simulink model "Fly_By_Wire_Functional_Architecture"  (R2024b)
settings: Solver=VariableStepAuto  StartTime=0.0  StopTime=10.0  RelTol=1e-3
settings Model: Creator=kmara  LastModifiedBy=annicenajafi

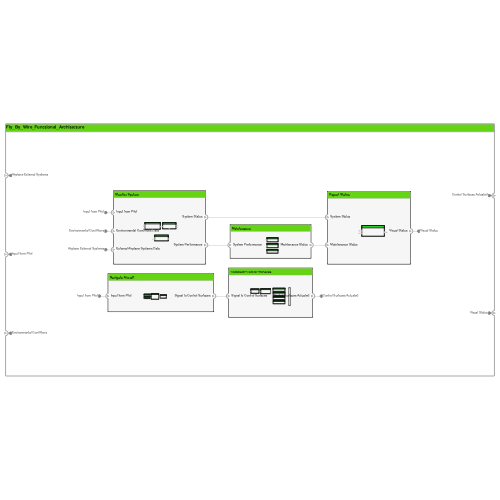
[thumbnail: Simulink's stored preview of the top-level diagram]
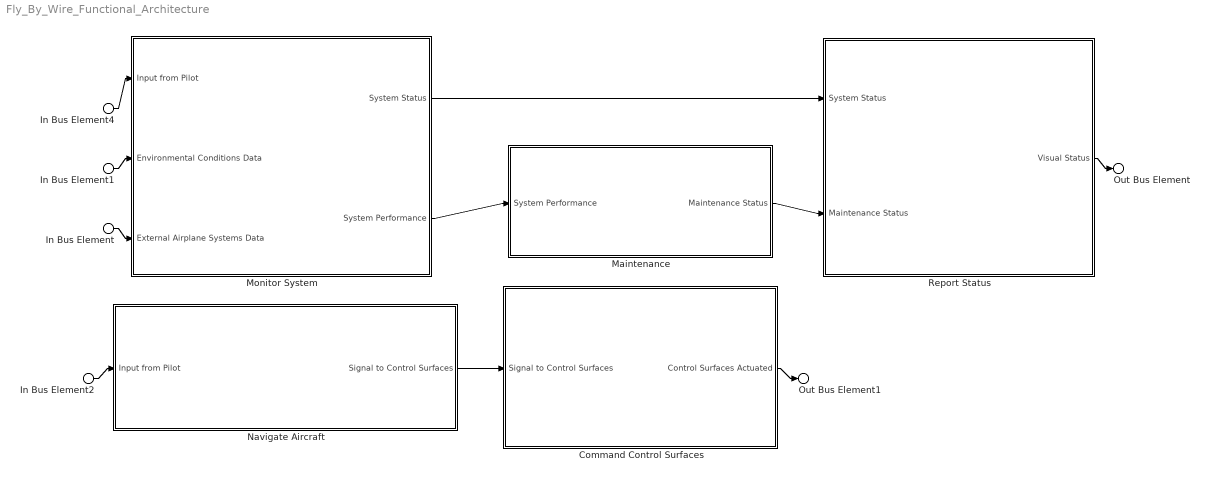
== system Fly_By_Wire_Functional_Architecture ==
  In Bus Element : Inport  PortName=Airplane External Systems
  In Bus Element2 : Inport  Port=2  PortName=Input from Pilot
  In Bus Element4 : Inport  Port=2  PortName=Input from Pilot
  In Bus Element1 : Inport  Port=3  PortName=Environmental Conditions
  Command Control Surfaces : Subsystem
      settings: PortSchema="{\"entries\":[{\"content\":{\"headerSize\":26,\"margin\":15,\"minimumSpacing\":25,\"sides\":[{\"content\":{\"connectorIds\":[\"In1\"]},\"type\":\"ConnectorPlacement.EquallySpacedRectSide\",\"uuid\":\"b623a921-0a01-4933-aa95-d281e4fd472d\"},{\"content\":{\"connectorIds\":[\"Out1\"],\"side\":\"RIGHT\"},\"type\":\"ConnectorPlacement.EquallySpacedRectSide\",\"uuid\":\"7949cc00-59a5-498d-8900-6268840cf223\"},{\"content\":{\"side\":\"TOP\"},\"type\":\"ConnectorPlacement.EquallySpacedRectSide\",\"uuid\":\"61a6df68-b8b8-47cf-a694-eae6da7c16c5\"}]},\"type\":\"ConnectorPlacement.EquallySpacedConnector\",\"uuid\":\"95d0e082-c8fd-4f2c-a7f4-dd74223482be\"}],\"packageUris\":[\"http://schema.mathworks.com/mf0/Connector/R2020b\"],\"version\":\"1.0\"}"
  Maintenance : Subsystem
      settings: PortSchema="{\"entries\":[{\"content\":{\"headerSize\":26,\"margin\":15,\"minimumSpacing\":25,\"sides\":[{\"content\":{\"connectorIds\":[\"In1\"]},\"type\":\"ConnectorPlacement.EquallySpacedRectSide\",\"uuid\":\"b623a921-0a01-4933-aa95-d281e4fd472d\"},{\"content\":{\"connectorIds\":[\"Out1\"],\"side\":\"RIGHT\"},\"type\":\"ConnectorPlacement.EquallySpacedRectSide\",\"uuid\":\"7949cc00-59a5-498d-8900-6268840cf223\"},{\"content\":{\"side\":\"TOP\"},\"type\":\"ConnectorPlacement.EquallySpacedRectSide\",\"uuid\":\"61a6df68-b8b8-47cf-a694-eae6da7c16c5\"},{\"content\":{\"side\":\"BOTTOM\"},\"type\":\"ConnectorPlacement.EquallySpacedRectSide\",\"uuid\":\"116ec3ef-5420-49c5-b776-94fc19793a99\"}]},\"type\":\"ConnectorPlacement.EquallySpacedConnector\",\"uuid\":\"95d0e082-c8fd-4f2c-a7f4-dd74223482be\"}],\"packageUris\":[\"http://schema.mathworks.com/mf0/Connector/R2020b\"],\"version\":\"1.0\"}"
  Monitor System : Subsystem
      settings: PortSchema="{\"entries\":[{\"content\":{\"headerSize\":26,\"margin\":15,\"minimumSpacing\":25,\"sides\":[{\"content\":{\"connectorIds\":[\"In1\",\"In2\",\"In3\"]},\"type\":\"ConnectorPlacement.EquallySpacedRectSide\",\"uuid\":\"ca232a45-352c-4197-a2f1-cf960b1c61e1\"},{\"content\":{\"connectorIds\":[\"Out2\",\"Out1\"],\"side\":\"RIGHT\"},\"type\":\"ConnectorPlacement.EquallySpacedRectSide\",\"uuid\":\"283c5dac-edd1-4fd8-b197-00019376217d\"},{\"content\":{\"side\":\"TOP\"},\"type\":\"ConnectorPlacement.EquallySpacedRectSide\",\"uuid\":\"42446a2b-1c27-4301-a80a-90130219a089\"},{\"content\":{\"side\":\"BOTTOM\"},\"type\":\"ConnectorPlacement.EquallySpacedRectSide\",\"uuid\":\"c57680a4-00c2-4754-bdc7-f63d5f759134\"}]},\"type\":\"ConnectorPlacement.EquallySpacedConnector\",\"uuid\":\"458bc52f-ed05-4f31-b732-8171eb2e03be\"}],\"packageUris\":[\"http://schema.mathworks.com/mf0/Connector/R2020b\"],\"version\":\"1.0\"}"
  Navigate Aircraft : Subsystem
      settings: PortSchema="{\"entries\":[{\"content\":{\"headerSize\":26,\"margin\":15,\"minimumSpacing\":25,\"sides\":[{\"content\":{\"connectorIds\":[\"In1\"]},\"type\":\"ConnectorPlacement.EquallySpacedRectSide\",\"uuid\":\"b623a921-0a01-4933-aa95-d281e4fd472d\"},{\"content\":{\"connectorIds\":[\"Out1\"],\"side\":\"RIGHT\"},\"type\":\"ConnectorPlacement.EquallySpacedRectSide\",\"uuid\":\"7949cc00-59a5-498d-8900-6268840cf223\"},{\"content\":{\"side\":\"TOP\"},\"type\":\"ConnectorPlacement.EquallySpacedRectSide\",\"uuid\":\"61a6df68-b8b8-47cf-a694-eae6da7c16c5\"}]},\"type\":\"ConnectorPlacement.EquallySpacedConnector\",\"uuid\":\"95d0e082-c8fd-4f2c-a7f4-dd74223482be\"}],\"packageUris\":[\"http://schema.mathworks.com/mf0/Connector/R2020b\"],\"version\":\"1.0\"}"
  Report Status : Subsystem
      settings: PortSchema="{\"entries\":[{\"content\":{\"headerSize\":26,\"margin\":15,\"minimumSpacing\":25,\"sides\":[{\"content\":{\"connectorIds\":[\"In2\",\"In1\"]},\"type\":\"ConnectorPlacement.EquallySpacedRectSide\",\"uuid\":\"ca232a45-352c-4197-a2f1-cf960b1c61e1\"},{\"content\":{\"connectorIds\":[\"Out1\"],\"side\":\"RIGHT\"},\"type\":\"ConnectorPlacement.EquallySpacedRectSide\",\"uuid\":\"283c5dac-edd1-4fd8-b197-00019376217d\"},{\"content\":{\"side\":\"TOP\"},\"type\":\"ConnectorPlacement.EquallySpacedRectSide\",\"uuid\":\"42446a2b-1c27-4301-a80a-90130219a089\"}]},\"type\":\"ConnectorPlacement.EquallySpacedConnector\",\"uuid\":\"458bc52f-ed05-4f31-b732-8171eb2e03be\"}],\"packageUris\":[\"http://schema.mathworks.com/mf0/Connector/R2020b\"],\"version\":\"1.0\"}"
  Out Bus Element1 : Outport  PortName=Control Surfaces Actuated
  Out Bus Element : Outport  Port=2  PortName=Visual Status
  wires:
  In Bus Element4/1 -> Monitor System/1(Input from Pilot)
  In Bus Element/1 -> Monitor System/3(External Airplane Systems Data)
  In Bus Element2/1 -> Navigate Aircraft/1(Input from Pilot)
  Navigate Aircraft/1(Signal to Control Surfaces) -> Command Control Surfaces/1(Signal to Control Surfaces)
  In Bus Element1/1 -> Monitor System/2(Environmental Conditions Data)
  Monitor System/1(System Performance) -> Maintenance/1(System Performance)
  Monitor System/2(System Status) -> Report Status/2(System Status)
  Maintenance/1(Maintenance Status) -> Report Status/1(Maintenance Status)
  Command Control Surfaces/1(Control Surfaces Actuated) -> Out Bus Element1/1
  Report Status/1(Visual Status) -> Out Bus Element/1

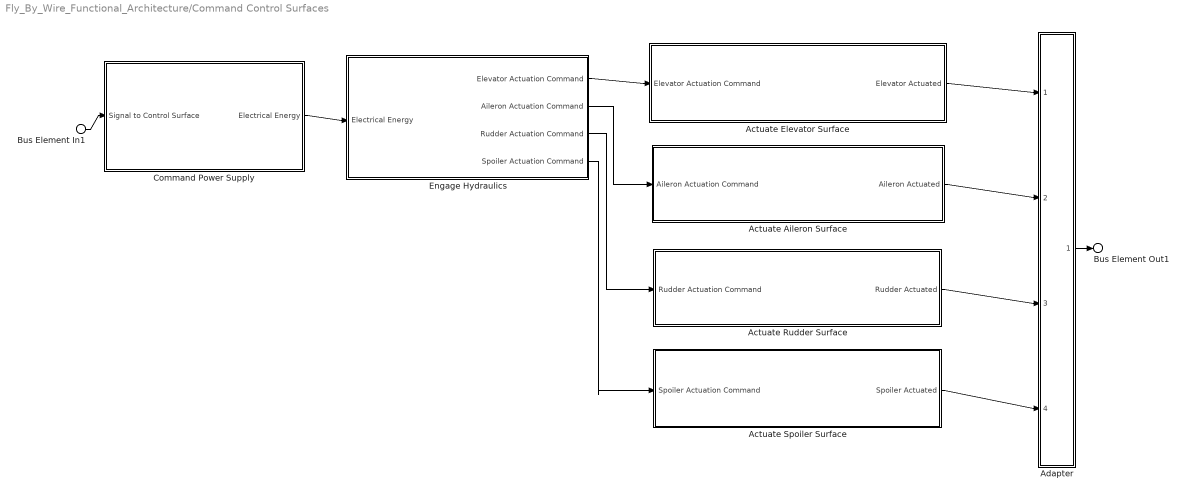
== system Fly_By_Wire_Functional_Architecture/Command Control Surfaces ==
  Bus Element In1 : Inport  PortName=Signal to Control Surfaces
  Actuate Aileron Surface : Subsystem
      settings: PortSchema="{\"entries\":[{\"content\":{\"headerSize\":26,\"margin\":15,\"minimumSpacing\":25,\"sides\":[{\"content\":{\"connectorIds\":[\"In1\"]},\"type\":\"ConnectorPlacement.EquallySpacedRectSide\",\"uuid\":\"b623a921-0a01-4933-aa95-d281e4fd472d\"},{\"content\":{\"connectorIds\":[\"Out1\"],\"side\":\"RIGHT\"},\"type\":\"ConnectorPlacement.EquallySpacedRectSide\",\"uuid\":\"7949cc00-59a5-498d-8900-6268840cf223\"},{\"content\":{\"side\":\"TOP\"},\"type\":\"ConnectorPlacement.EquallySpacedRectSide\",\"uuid\":\"61a6df68-b8b8-47cf-a694-eae6da7c16c5\"}]},\"type\":\"ConnectorPlacement.EquallySpacedConnector\",\"uuid\":\"95d0e082-c8fd-4f2c-a7f4-dd74223482be\"}],\"packageUris\":[\"http://schema.mathworks.com/mf0/Connector/R2020b\"],\"version\":\"1.0\"}"
  Actuate Elevator Surface : Subsystem
      settings: PortSchema="{\"entries\":[{\"content\":{\"headerSize\":26,\"margin\":15,\"minimumSpacing\":25,\"sides\":[{\"content\":{\"connectorIds\":[\"In1\"]},\"type\":\"ConnectorPlacement.EquallySpacedRectSide\",\"uuid\":\"b623a921-0a01-4933-aa95-d281e4fd472d\"},{\"content\":{\"connectorIds\":[\"Out1\"],\"side\":\"RIGHT\"},\"type\":\"ConnectorPlacement.EquallySpacedRectSide\",\"uuid\":\"7949cc00-59a5-498d-8900-6268840cf223\"},{\"content\":{\"side\":\"TOP\"},\"type\":\"ConnectorPlacement.EquallySpacedRectSide\",\"uuid\":\"61a6df68-b8b8-47cf-a694-eae6da7c16c5\"}]},\"type\":\"ConnectorPlacement.EquallySpacedConnector\",\"uuid\":\"95d0e082-c8fd-4f2c-a7f4-dd74223482be\"}],\"packageUris\":[\"http://schema.mathworks.com/mf0/Connector/R2020b\"],\"version\":\"1.0\"}"
  Actuate Rudder Surface : Subsystem
      settings: PortSchema="{\"entries\":[{\"content\":{\"headerSize\":26,\"margin\":15,\"minimumSpacing\":25,\"sides\":[{\"content\":{\"connectorIds\":[\"In1\"]},\"type\":\"ConnectorPlacement.EquallySpacedRectSide\",\"uuid\":\"b623a921-0a01-4933-aa95-d281e4fd472d\"},{\"content\":{\"connectorIds\":[\"Out1\"],\"side\":\"RIGHT\"},\"type\":\"ConnectorPlacement.EquallySpacedRectSide\",\"uuid\":\"7949cc00-59a5-498d-8900-6268840cf223\"},{\"content\":{\"side\":\"TOP\"},\"type\":\"ConnectorPlacement.EquallySpacedRectSide\",\"uuid\":\"61a6df68-b8b8-47cf-a694-eae6da7c16c5\"}]},\"type\":\"ConnectorPlacement.EquallySpacedConnector\",\"uuid\":\"95d0e082-c8fd-4f2c-a7f4-dd74223482be\"}],\"packageUris\":[\"http://schema.mathworks.com/mf0/Connector/R2020b\"],\"version\":\"1.0\"}"
  Actuate Spoiler Surface : Subsystem
      settings: PortSchema="{\"entries\":[{\"content\":{\"headerSize\":26,\"margin\":15,\"minimumSpacing\":25,\"sides\":[{\"content\":{\"connectorIds\":[\"In1\"]},\"type\":\"ConnectorPlacement.EquallySpacedRectSide\",\"uuid\":\"b623a921-0a01-4933-aa95-d281e4fd472d\"},{\"content\":{\"connectorIds\":[\"Out1\"],\"side\":\"RIGHT\"},\"type\":\"ConnectorPlacement.EquallySpacedRectSide\",\"uuid\":\"7949cc00-59a5-498d-8900-6268840cf223\"},{\"content\":{\"side\":\"TOP\"},\"type\":\"ConnectorPlacement.EquallySpacedRectSide\",\"uuid\":\"61a6df68-b8b8-47cf-a694-eae6da7c16c5\"}]},\"type\":\"ConnectorPlacement.EquallySpacedConnector\",\"uuid\":\"95d0e082-c8fd-4f2c-a7f4-dd74223482be\"}],\"packageUris\":[\"http://schema.mathworks.com/mf0/Connector/R2020b\"],\"version\":\"1.0\"}"
  Adapter : Subsystem
      settings: PortSchema="{\"entries\":[{\"content\":{\"margin\":10,\"minimumSpacing\":15,\"sides\":[{\"content\":{\"connectorIds\":[\"In1\",\"In2\",\"In3\",\"In4\"]},\"type\":\"ConnectorPlacement.EquallySpacedRectSide\",\"uuid\":\"e46bc7ad-37e4-4738-9cce-4544dbd88a61\"},{\"content\":{\"connectorIds\":[\"Out1\"],\"side\":\"RIGHT\"},\"type\":\"ConnectorPlacement.EquallySpacedRectSide\",\"uuid\":\"8c580fa9-ae3a-4a2b-b582-24b4f761d043\"},{\"content\":{\"side\":\"TOP\"},\"type\":\"ConnectorPlacement.EquallySpacedRectSide\",\"uuid\":\"ae7dedc0-cfa3-425e-8c68-3d421b20d73f\"},{\"content\":{\"side\":\"BOTTOM\"},\"type\":\"ConnectorPlacement.EquallySpacedRectSide\",\"uuid\":\"1952df18-3b35-4b06-af68-5997b372901e\"}]},\"type\":\"ConnectorPlacement.EquallySpacedConnector\",\"uuid\":\"f6cfd067-dcc4-463f-810a-2a6848ea874f\"}],\"packageUris\":[\"http://schema.mathworks.com/mf0/Connector/R2020b\"],\"version\":\"1.0\"}"
  Command Power Supply : Subsystem
      settings: PortSchema="{\"entries\":[{\"content\":{\"headerSize\":26,\"margin\":15,\"minimumSpacing\":25,\"sides\":[{\"content\":{\"connectorIds\":[\"In1\"]},\"type\":\"ConnectorPlacement.EquallySpacedRectSide\",\"uuid\":\"b623a921-0a01-4933-aa95-d281e4fd472d\"},{\"content\":{\"connectorIds\":[\"Out1\"],\"side\":\"RIGHT\"},\"type\":\"ConnectorPlacement.EquallySpacedRectSide\",\"uuid\":\"7949cc00-59a5-498d-8900-6268840cf223\"},{\"content\":{\"side\":\"TOP\"},\"type\":\"ConnectorPlacement.EquallySpacedRectSide\",\"uuid\":\"61a6df68-b8b8-47cf-a694-eae6da7c16c5\"}]},\"type\":\"ConnectorPlacement.EquallySpacedConnector\",\"uuid\":\"95d0e082-c8fd-4f2c-a7f4-dd74223482be\"}],\"packageUris\":[\"http://schema.mathworks.com/mf0/Connector/R2020b\"],\"version\":\"1.0\"}"
  Engage Hydraulics : Subsystem
      settings: PortSchema="{\"entries\":[{\"content\":{\"headerSize\":26,\"margin\":15,\"minimumSpacing\":25,\"sides\":[{\"content\":{\"connectorIds\":[\"In1\"]},\"type\":\"ConnectorPlacement.EquallySpacedRectSide\",\"uuid\":\"b623a921-0a01-4933-aa95-d281e4fd472d\"},{\"content\":{\"connectorIds\":[\"Out1\",\"Out2\",\"Out3\",\"Out4\"],\"side\":\"RIGHT\"},\"type\":\"ConnectorPlacement.EquallySpacedRectSide\",\"uuid\":\"7949cc00-59a5-498d-8900-6268840cf223\"},{\"content\":{\"side\":\"TOP\"},\"type\":\"ConnectorPlacement.EquallySpacedRectSide\",\"uuid\":\"61a6df68-b8b8-47cf-a694-eae6da7c16c5\"}]},\"type\":\"ConnectorPlacement.EquallySpacedConnector\",\"uuid\":\"95d0e082-c8fd-4f2c-a7f4-dd74223482be\"}],\"packageUris\":[\"http://schema.mathworks.com/mf0/Connector/R2020b\"],\"version\":\"1.0\"}"
  Bus Element Out1 : Outport  PortName=Control Surfaces Actuated
  wires:
  Actuate Aileron Surface/1(Aileron Actuated) -> Adapter/2(Aileron Actuated)
  Bus Element In1/1 -> Command Power Supply/1(Signal to Control Surface)
  Adapter/1(Control Surfaces Actuated) -> Bus Element Out1/1
  Engage Hydraulics/1(Elevator Actuation Command) -> Actuate Elevator Surface/1(Elevator Actuation Command)
  Command Power Supply/1(Electrical Energy) -> Engage Hydraulics/1(Electrical Energy)
  Engage Hydraulics/2(Aileron Actuation Command) -> Actuate Aileron Surface/1(Aileron Actuation Command)
  Engage Hydraulics/4(" Spoiler Actuation Command") -> Actuate Spoiler Surface/1(" Spoiler Actuation Command")
  Engage Hydraulics/3(" Rudder Actuation Command") -> Actuate Rudder Surface/1(" Rudder Actuation Command")
  Actuate Elevator Surface/1(Elevator Actuated) -> Adapter/1(Elevator Actuated)
  Actuate Rudder Surface/1(Rudder Actuated) -> Adapter/3(Rudder Actuated)
  Actuate Spoiler Surface/1(Spoiler Actuated) -> Adapter/4(Spoiler Actuated)

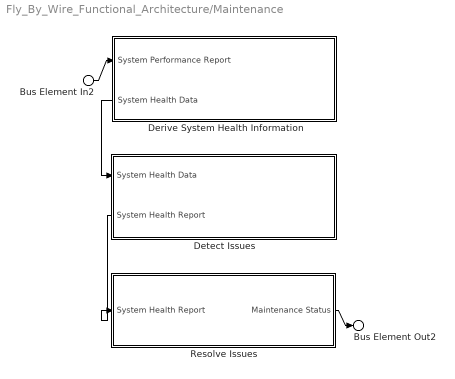
== system Fly_By_Wire_Functional_Architecture/Maintenance ==
  Bus Element In2 : Inport  PortName=System Performance
  Derive System Health Information : Subsystem
      settings: PortSchema="{\"entries\":[{\"content\":{\"headerSize\":26,\"margin\":15,\"minimumSpacing\":25,\"sides\":[{\"content\":{\"connectorIds\":[\"In1\",\"Out1\"]},\"type\":\"ConnectorPlacement.EquallySpacedRectSide\",\"uuid\":\"b623a921-0a01-4933-aa95-d281e4fd472d\"},{\"content\":{\"side\":\"RIGHT\"},\"type\":\"ConnectorPlacement.EquallySpacedRectSide\",\"uuid\":\"7949cc00-59a5-498d-8900-6268840cf223\"},{\"content\":{\"side\":\"TOP\"},\"type\":\"ConnectorPlacement.EquallySpacedRectSide\",\"uuid\":\"61a6df68-b8b8-47cf-a694-eae6da7c16c5\"},{\"content\":{\"side\":\"BOTTOM\"},\"type\":\"ConnectorPlacement.EquallySpacedRectSide\",\"uuid\":\"513e8f81-150e-4fea-8a25-5ca370c72a01\"}]},\"type\":\"ConnectorPlacement.EquallySpacedConnector\",\"uuid\":\"95d0e082-c8fd-4f2c-a7f4-dd74223482be\"}],\"packageUris\":[\"http://schema.mathworks.com/mf0/Connector/R2020b\"],\"version\":\"1.0\"}"
  Detect Issues : Subsystem
      settings: PortSchema="{\"entries\":[{\"content\":{\"headerSize\":26,\"margin\":15,\"minimumSpacing\":25,\"sides\":[{\"content\":{\"connectorIds\":[\"In1\",\"Out1\"]},\"type\":\"ConnectorPlacement.EquallySpacedRectSide\",\"uuid\":\"b623a921-0a01-4933-aa95-d281e4fd472d\"},{\"content\":{\"side\":\"RIGHT\"},\"type\":\"ConnectorPlacement.EquallySpacedRectSide\",\"uuid\":\"7949cc00-59a5-498d-8900-6268840cf223\"},{\"content\":{\"side\":\"TOP\"},\"type\":\"ConnectorPlacement.EquallySpacedRectSide\",\"uuid\":\"61a6df68-b8b8-47cf-a694-eae6da7c16c5\"},{\"content\":{\"side\":\"BOTTOM\"},\"type\":\"ConnectorPlacement.EquallySpacedRectSide\",\"uuid\":\"aee534c5-854d-492b-acf9-b9cae6f63452\"}]},\"type\":\"ConnectorPlacement.EquallySpacedConnector\",\"uuid\":\"95d0e082-c8fd-4f2c-a7f4-dd74223482be\"}],\"packageUris\":[\"http://schema.mathworks.com/mf0/Connector/R2020b\"],\"version\":\"1.0\"}"
  Resolve Issues : Subsystem
      settings: PortSchema="{\"entries\":[{\"content\":{\"headerSize\":26,\"margin\":15,\"minimumSpacing\":25,\"sides\":[{\"content\":{\"connectorIds\":[\"In1\"]},\"type\":\"ConnectorPlacement.EquallySpacedRectSide\",\"uuid\":\"b623a921-0a01-4933-aa95-d281e4fd472d\"},{\"content\":{\"connectorIds\":[\"Out1\"],\"side\":\"RIGHT\"},\"type\":\"ConnectorPlacement.EquallySpacedRectSide\",\"uuid\":\"7949cc00-59a5-498d-8900-6268840cf223\"},{\"content\":{\"side\":\"TOP\"},\"type\":\"ConnectorPlacement.EquallySpacedRectSide\",\"uuid\":\"61a6df68-b8b8-47cf-a694-eae6da7c16c5\"},{\"content\":{\"side\":\"BOTTOM\"},\"type\":\"ConnectorPlacement.EquallySpacedRectSide\",\"uuid\":\"19c685d9-7558-4e2a-bcd3-063abede9b38\"}]},\"type\":\"ConnectorPlacement.EquallySpacedConnector\",\"uuid\":\"95d0e082-c8fd-4f2c-a7f4-dd74223482be\"}],\"packageUris\":[\"http://schema.mathworks.com/mf0/Connector/R2020b\"],\"version\":\"1.0\"}"
  Bus Element Out2 : Outport  PortName=Maintenance Status
  wires:
  Derive System Health Information/1(System Health Data) -> Detect Issues/1(System Health Data)
  Detect Issues/1(System Health Report) -> Resolve Issues/1(System Health Report)
  Bus Element In2/1 -> Derive System Health Information/1(System Performance Report)
  Resolve Issues/1(Maintenance Status) -> Bus Element Out2/1

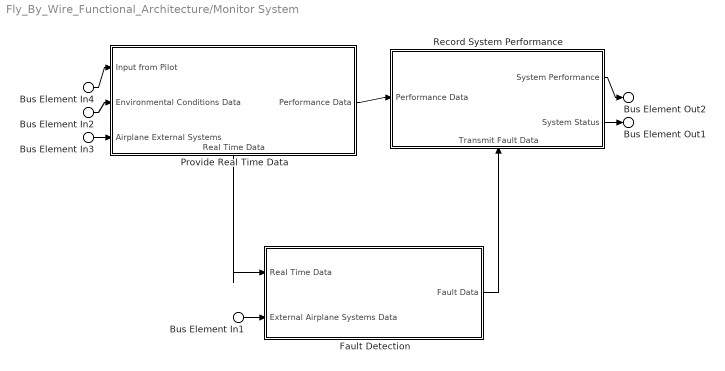
== system Fly_By_Wire_Functional_Architecture/Monitor System ==
  Bus Element In4 : Inport  PortName=Input from Pilot
  Bus Element In2 : Inport  Port=2  PortName=Environmental Conditions Data
  Bus Element In1 : Inport  Port=3  PortName=External Airplane Systems Data
  Bus Element In3 : Inport  Port=3  PortName=External Airplane Systems Data
  Fault Detection : Subsystem
      settings: PortSchema="{\"entries\":[{\"content\":{\"headerSize\":26,\"margin\":15,\"minimumSpacing\":25,\"sides\":[{\"content\":{\"connectorIds\":[\"In1\",\"In2\"]},\"type\":\"ConnectorPlacement.EquallySpacedRectSide\",\"uuid\":\"7c02a101-dcdb-4ce7-aa42-618b1352dc14\"},{\"content\":{\"connectorIds\":[\"Out1\"],\"side\":\"RIGHT\"},\"type\":\"ConnectorPlacement.EquallySpacedRectSide\",\"uuid\":\"7a5c8ca0-4377-40e0-b018-2d4752105c97\"},{\"content\":{\"side\":\"TOP\"},\"type\":\"ConnectorPlacement.EquallySpacedRectSide\",\"uuid\":\"1a585cfa-94cd-4fa4-8da7-05bff58353c8\"}]},\"type\":\"ConnectorPlacement.EquallySpacedConnector\",\"uuid\":\"b5a72803-1929-44a1-ac0b-19b19b30c1d3\"}],\"packageUris\":[\"http://schema.mathworks.com/mf0/Connector/R2020b\"],\"version\":\"1.0\"}"
  Provide Real Time Data : Subsystem
      settings: PortSchema="{\"entries\":[{\"content\":{\"headerSize\":26,\"margin\":15,\"minimumSpacing\":25,\"sides\":[{\"content\":{\"connectorIds\":[\"In1\",\"In2\",\"In3\"]},\"type\":\"ConnectorPlacement.EquallySpacedRectSide\",\"uuid\":\"7c02a101-dcdb-4ce7-aa42-618b1352dc14\"},{\"content\":{\"connectorIds\":[\"Out2\"],\"side\":\"RIGHT\"},\"type\":\"ConnectorPlacement.EquallySpacedRectSide\",\"uuid\":\"7a5c8ca0-4377-40e0-b018-2d4752105c97\"},{\"content\":{\"side\":\"TOP\"},\"type\":\"ConnectorPlacement.EquallySpacedRectSide\",\"uuid\":\"1a585cfa-94cd-4fa4-8da7-05bff58353c8\"},{\"content\":{\"connectorIds\":[\"Out1\"],\"side\":\"BOTTOM\"},\"type\":\"ConnectorPlacement.EquallySpacedRectSide\",\"uuid\":\"75dcf8ad-400d-4ec8-8030-4d83993c479e\"}]},\"type\":\"ConnectorPlacement.EquallySpacedConnector\",\"uuid\":\"b5a72803-1929-44a1-ac0b-19b19b30c1d3\"}],\"packageUris\":[\"http://schema.mathworks.com/mf0/Connector/R2020b\"],\"version\":\"1.0\"}"
  Record System Performance : Subsystem
      settings: PortSchema="{\"entries\":[{\"content\":{\"headerSize\":26,\"margin\":15,\"minimumSpacing\":25,\"sides\":[{\"content\":{\"connectorIds\":[\"In2\"]},\"type\":\"ConnectorPlacement.EquallySpacedRectSide\",\"uuid\":\"7c02a101-dcdb-4ce7-aa42-618b1352dc14\"},{\"content\":{\"connectorIds\":[\"Out1\",\"Out2\"],\"side\":\"RIGHT\"},\"type\":\"ConnectorPlacement.EquallySpacedRectSide\",\"uuid\":\"7a5c8ca0-4377-40e0-b018-2d4752105c97\"},{\"content\":{\"side\":\"TOP\"},\"type\":\"ConnectorPlacement.EquallySpacedRectSide\",\"uuid\":\"1a585cfa-94cd-4fa4-8da7-05bff58353c8\"},{\"content\":{\"connectorIds\":[\"In1\"],\"side\":\"BOTTOM\"},\"type\":\"ConnectorPlacement.EquallySpacedRectSide\",\"uuid\":\"d82d0e77-3fde-48c0-9f05-495eb32de877\"}]},\"type\":\"ConnectorPlacement.EquallySpacedConnector\",\"uuid\":\"b5a72803-1929-44a1-ac0b-19b19b30c1d3\"}],\"packageUris\":[\"http://schema.mathworks.com/mf0/Connector/R2020b\"],\"version\":\"1.0\"}"
  Bus Element Out2 : Outport  PortName=System Performance
  Bus Element Out1 : Outport  Port=2  PortName=System Status
  wires:
  Bus Element In1/1 -> Fault Detection/2(External Airplane Systems Data)
  Bus Element In2/1 -> Provide Real Time Data/2(Environmental Conditions Data)
  Bus Element In3/1 -> Provide Real Time Data/3(Airplane External Systems)
  Provide Real Time Data/2(Performance Data) -> Record System Performance/2(Performance Data)
  Fault Detection/1(Fault Data) -> Record System Performance/1(Transmit Fault Data)
  Provide Real Time Data/1(Real Time Data) -> Fault Detection/1(Real Time Data)
  Bus Element In4/1 -> Provide Real Time Data/1(Input from Pilot)
  Record System Performance/1(System Performance) -> Bus Element Out2/1
  Record System Performance/2(System Status) -> Bus Element Out1/1

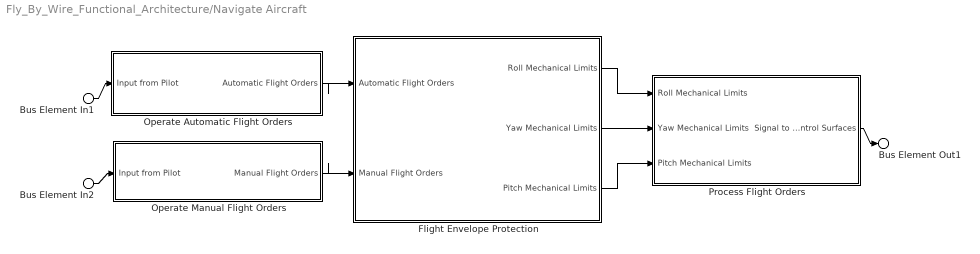
== system Fly_By_Wire_Functional_Architecture/Navigate Aircraft ==
  Bus Element In1 : Inport  PortName=Input from Pilot
  Bus Element In2 : Inport  PortName=Input from Pilot
  Flight Envelope Protection : Subsystem
      settings: PortSchema="{\"entries\":[{\"content\":{\"headerSize\":26,\"margin\":15,\"minimumSpacing\":25,\"sides\":[{\"content\":{\"connectorIds\":[\"In1\",\"In2\"]},\"type\":\"ConnectorPlacement.EquallySpacedRectSide\",\"uuid\":\"b623a921-0a01-4933-aa95-d281e4fd472d\"},{\"content\":{\"connectorIds\":[\"Out3\",\"Out2\",\"Out1\"],\"side\":\"RIGHT\"},\"type\":\"ConnectorPlacement.EquallySpacedRectSide\",\"uuid\":\"7949cc00-59a5-498d-8900-6268840cf223\"},{\"content\":{\"side\":\"TOP\"},\"type\":\"ConnectorPlacement.EquallySpacedRectSide\",\"uuid\":\"61a6df68-b8b8-47cf-a694-eae6da7c16c5\"},{\"content\":{\"side\":\"BOTTOM\"},\"type\":\"ConnectorPlacement.EquallySpacedRectSide\",\"uuid\":\"54f3ef6f-1ef2-4e47-9861-ed87ae28a6bb\"}]},\"type\":\"ConnectorPlacement.EquallySpacedConnector\",\"uuid\":\"95d0e082-c8fd-4f2c-a7f4-dd74223482be\"}],\"packageUris\":[\"http://schema.mathworks.com/mf0/Connector/R2020b\"],\"version\":\"1.0\"}"
  Operate Automatic Flight Orders : Subsystem
      settings: PortSchema="{\"entries\":[{\"content\":{\"headerSize\":26,\"margin\":15,\"minimumSpacing\":25,\"sides\":[{\"content\":{\"connectorIds\":[\"In1\"]},\"type\":\"ConnectorPlacement.EquallySpacedRectSide\",\"uuid\":\"ca232a45-352c-4197-a2f1-cf960b1c61e1\"},{\"content\":{\"connectorIds\":[\"Out1\"],\"side\":\"RIGHT\"},\"type\":\"ConnectorPlacement.EquallySpacedRectSide\",\"uuid\":\"283c5dac-edd1-4fd8-b197-00019376217d\"},{\"content\":{\"side\":\"TOP\"},\"type\":\"ConnectorPlacement.EquallySpacedRectSide\",\"uuid\":\"42446a2b-1c27-4301-a80a-90130219a089\"}]},\"type\":\"ConnectorPlacement.EquallySpacedConnector\",\"uuid\":\"458bc52f-ed05-4f31-b732-8171eb2e03be\"}],\"packageUris\":[\"http://schema.mathworks.com/mf0/Connector/R2020b\"],\"version\":\"1.0\"}"
  Operate Manual Flight Orders : Subsystem
      settings: PortSchema="{\"entries\":[{\"content\":{\"headerSize\":26,\"margin\":15,\"minimumSpacing\":25,\"sides\":[{\"content\":{\"connectorIds\":[\"In1\"]},\"type\":\"ConnectorPlacement.EquallySpacedRectSide\",\"uuid\":\"ca232a45-352c-4197-a2f1-cf960b1c61e1\"},{\"content\":{\"connectorIds\":[\"Out1\"],\"side\":\"RIGHT\"},\"type\":\"ConnectorPlacement.EquallySpacedRectSide\",\"uuid\":\"283c5dac-edd1-4fd8-b197-00019376217d\"},{\"content\":{\"side\":\"TOP\"},\"type\":\"ConnectorPlacement.EquallySpacedRectSide\",\"uuid\":\"42446a2b-1c27-4301-a80a-90130219a089\"}]},\"type\":\"ConnectorPlacement.EquallySpacedConnector\",\"uuid\":\"458bc52f-ed05-4f31-b732-8171eb2e03be\"}],\"packageUris\":[\"http://schema.mathworks.com/mf0/Connector/R2020b\"],\"version\":\"1.0\"}"
  Process Flight Orders : Subsystem
      settings: PortSchema="{\"entries\":[{\"content\":{\"headerSize\":26,\"margin\":15,\"minimumSpacing\":25,\"sides\":[{\"content\":{\"connectorIds\":[\"In1\",\"In2\",\"In3\"]},\"type\":\"ConnectorPlacement.EquallySpacedRectSide\",\"uuid\":\"b623a921-0a01-4933-aa95-d281e4fd472d\"},{\"content\":{\"connectorIds\":[\"Out1\"],\"side\":\"RIGHT\"},\"type\":\"ConnectorPlacement.EquallySpacedRectSide\",\"uuid\":\"7949cc00-59a5-498d-8900-6268840cf223\"},{\"content\":{\"side\":\"TOP\"},\"type\":\"ConnectorPlacement.EquallySpacedRectSide\",\"uuid\":\"61a6df68-b8b8-47cf-a694-eae6da7c16c5\"},{\"content\":{\"side\":\"BOTTOM\"},\"type\":\"ConnectorPlacement.EquallySpacedRectSide\",\"uuid\":\"acb69559-d835-40d8-9946-e225c1a09b2a\"}]},\"type\":\"ConnectorPlacement.EquallySpacedConnector\",\"uuid\":\"95d0e082-c8fd-4f2c-a7f4-dd74223482be\"}],\"packageUris\":[\"http://schema.mathworks.com/mf0/Connector/R2020b\"],\"version\":\"1.0\"}"
  Bus Element Out1 : Outport  PortName=Signal to Control Surfaces
  wires:
  Bus Element In2/1 -> Operate Manual Flight Orders/1(Input from Pilot)
  Bus Element In1/1 -> Operate Automatic Flight Orders/1(Input from Pilot)
  Flight Envelope Protection/1(Pitch Mechanical Limits) -> Process Flight Orders/3(Pitch Mechanical Limits)
  Flight Envelope Protection/2(Yaw Mechanical Limits) -> Process Flight Orders/2(Yaw Mechanical Limits)
  Flight Envelope Protection/3(Roll Mechanical Limits) -> Process Flight Orders/1(Roll Mechanical Limits)
  Operate Automatic Flight Orders/1(Automatic Flight Orders) -> Flight Envelope Protection/1(Automatic Flight Orders)
  Process Flight Orders/1(Signal to Control Surfaces) -> Bus Element Out1/1
  Operate Manual Flight Orders/1(Manual Flight Orders) -> Flight Envelope Protection/2(Manual Flight Orders)

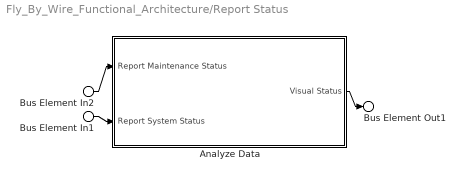
== system Fly_By_Wire_Functional_Architecture/Report Status ==
  Bus Element In2 : Inport  PortName=Maintenance Status
  Bus Element In1 : Inport  Port=2  PortName=System Status
  Analyze Data : Subsystem
      settings: PortSchema="{\"entries\":[{\"content\":{\"headerSize\":26,\"margin\":15,\"minimumSpacing\":25,\"sides\":[{\"content\":{\"connectorIds\":[\"In1\",\"In2\"]},\"type\":\"ConnectorPlacement.EquallySpacedRectSide\",\"uuid\":\"7c02a101-dcdb-4ce7-aa42-618b1352dc14\"},{\"content\":{\"connectorIds\":[\"Out1\"],\"side\":\"RIGHT\"},\"type\":\"ConnectorPlacement.EquallySpacedRectSide\",\"uuid\":\"7a5c8ca0-4377-40e0-b018-2d4752105c97\"},{\"content\":{\"side\":\"TOP\"},\"type\":\"ConnectorPlacement.EquallySpacedRectSide\",\"uuid\":\"1a585cfa-94cd-4fa4-8da7-05bff58353c8\"}]},\"type\":\"ConnectorPlacement.EquallySpacedConnector\",\"uuid\":\"b5a72803-1929-44a1-ac0b-19b19b30c1d3\"}],\"packageUris\":[\"http://schema.mathworks.com/mf0/Connector/R2020b\"],\"version\":\"1.0\"}"
  Bus Element Out1 : Outport  PortName=Visual Status
  wires:
  Bus Element In2/1 -> Analyze Data/1(Report Maintenance Status)
  Bus Element In1/1 -> Analyze Data/2(Report System Status)
  Analyze Data/1(Visual Status) -> Bus Element Out1/1

== system Fly_By_Wire_Functional_Architecture/Command Control Surfaces/Actuate Aileron Surface ==
  Bus Element In1 : Inport  PortName=Aileron Actuation Command
  Bus Element Out1 : Outport  PortName=Aileron Actuated

== system Fly_By_Wire_Functional_Architecture/Command Control Surfaces/Actuate Elevator Surface ==
  Bus Element In1 : Inport  PortName=Elevator Actuation Command
  Bus Element Out1 : Outport  PortName=Elevator Actuated

== system Fly_By_Wire_Functional_Architecture/Command Control Surfaces/Actuate Rudder Surface ==
  Bus Element In1 : Inport  PortName=Rudder Actuation Command
  Bus Element Out1 : Outport  PortName=Rudder Actuated

== system Fly_By_Wire_Functional_Architecture/Command Control Surfaces/Actuate Spoiler Surface ==
  Bus Element In1 : Inport  PortName=Spoiler Actuation Command
  Bus Element Out1 : Outport  PortName=Spoiler Actuated

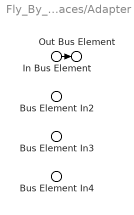
== system Fly_By_Wire_Functional_Architecture/Command Control Surfaces/Adapter ==
  In Bus Element : Inport  PortName=Elevator Actuated
  Bus Element In2 : Inport  Port=2  PortName=Aileron Actuated
  Bus Element In3 : Inport  Port=3  PortName=Rudder Actuated
  Bus Element In4 : Inport  Port=4  PortName=Spoiler Actuated
  Out Bus Element : Outport  PortName=Control Surfaces Actuated
  wires:
  In Bus Element/1 -> Out Bus Element/1

== system Fly_By_Wire_Functional_Architecture/Command Control Surfaces/Command Power Supply ==
  Bus Element In1 : Inport  PortName=Signal to Control Surface
  Bus Element Out1 : Outport  PortName=Electrical Energy

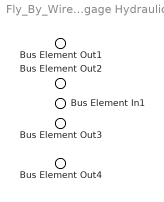
== system Fly_By_Wire_Functional_Architecture/Command Control Surfaces/Engage Hydraulics ==
  Bus Element In1 : Inport  PortName=Electrical Energy
  Bus Element Out1 : Outport  PortName=Elevator Actuation Command
  Bus Element Out2 : Outport  Port=2  PortName=Aileron Actuation Command
  Bus Element Out3 : Outport  Port=3  PortName=Rudder Actuation Command
  Bus Element Out4 : Outport  Port=4  PortName=Spoiler Actuation Command

== system Fly_By_Wire_Functional_Architecture/Maintenance/Derive System Health Information ==
  Bus Element In2 : Inport  PortName=System Performance Report
  Bus Element Out1 : Outport  PortName=System Health Data

== system Fly_By_Wire_Functional_Architecture/Maintenance/Detect Issues ==
  Bus Element In1 : Inport  PortName=System Health Data
  Bus Element Out1 : Outport  PortName=System Health Report

== system Fly_By_Wire_Functional_Architecture/Maintenance/Resolve Issues ==
  Bus Element In1 : Inport  PortName=System Health Report
  Bus Element Out1 : Outport  PortName=Maintenance Status

== system Fly_By_Wire_Functional_Architecture/Monitor System/Fault Detection ==
  Bus Element In2 : Inport  PortName=Real Time Data
  Bus Element In1 : Inport  Port=2  PortName=External Airplane Systems Data
  Bus Element Out1 : Outport  PortName=Fault Data

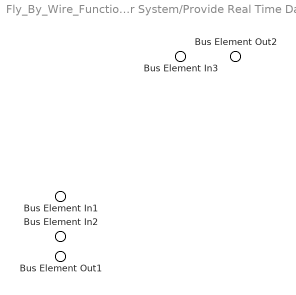
== system Fly_By_Wire_Functional_Architecture/Monitor System/Provide Real Time Data ==
  Bus Element In3 : Inport  PortName=Input from Pilot
  Bus Element In1 : Inport  Port=2  PortName=Environmental Conditions Data
  Bus Element In2 : Inport  Port=3  PortName=Airplane External Systems
  Bus Element Out2 : Outport  PortName=Real Time Data
  Bus Element Out1 : Outport  Port=2  PortName=Performance Data

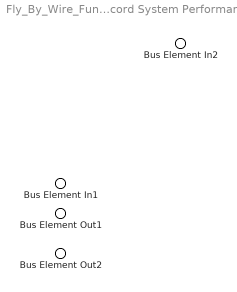
== system Fly_By_Wire_Functional_Architecture/Monitor System/Record System Performance ==
  Bus Element In2 : Inport  PortName=Transmit Fault Data
  Bus Element In1 : Inport  Port=2  PortName=Performance Data
  Bus Element Out1 : Outport  PortName=System Performance
  Bus Element Out2 : Outport  Port=2  PortName=System Status

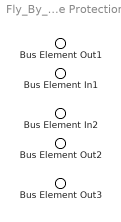
== system Fly_By_Wire_Functional_Architecture/Navigate Aircraft/Flight Envelope Protection ==
  Bus Element In1 : Inport  PortName=Automatic Flight Orders
  Bus Element In2 : Inport  Port=2  PortName=Manual Flight Orders
  Bus Element Out1 : Outport  PortName=Pitch Mechanical Limits
  Bus Element Out2 : Outport  Port=2  PortName=Yaw Mechanical Limits
  Bus Element Out3 : Outport  Port=3  PortName=Roll Mechanical Limits

== system Fly_By_Wire_Functional_Architecture/Navigate Aircraft/Operate Automatic Flight Orders ==
  Bus Element In1 : Inport  PortName=Input from Pilot
  Bus Element Out1 : Outport  PortName=Automatic Flight Orders

== system Fly_By_Wire_Functional_Architecture/Navigate Aircraft/Operate Manual Flight Orders ==
  Bus Element In1 : Inport  PortName=Input from Pilot
  Bus Element Out1 : Outport  PortName=Manual Flight Orders

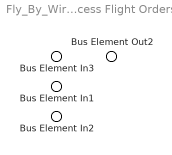
== system Fly_By_Wire_Functional_Architecture/Navigate Aircraft/Process Flight Orders ==
  Bus Element In2 : Inport  PortName=Roll Mechanical Limits
  Bus Element In1 : Inport  Port=2  PortName=Yaw Mechanical Limits
  Bus Element In3 : Inport  Port=3  PortName=Pitch Mechanical Limits
  Bus Element Out2 : Outport  PortName=Signal to Control Surfaces

== system Fly_By_Wire_Functional_Architecture/Report Status/Analyze Data ==
  Bus Element In1 : Inport  PortName=Report Maintenance Status
  Bus Element In2 : Inport  Port=2  PortName=Report System Status
  Bus Element Out1 : Outport  PortName=Visual Status
